simulink model "simulator"  (Simulink 7.3)
settings: Solver=ode1  SolverMode=SingleTasking  StartTime=0.0  StopTime=4  FixedStep=0.001  RelTol=1e-3
values from neighbouring files (symbols this model uses):
  Beq = 0.0015*6    (= 0.009)    [Sve ikad.m]    (also in matlab.mat = 0.0075)
  Eff_G = 0.9    [Sve ikad.m]    (also in matlab.mat)
  Eff_M = 0.69    [Sve ikad.m]    (also in matlab.mat)
  Jeq = 2e-3    (= 0.002)    [Sve ikad.m]    (also in matlab.mat)
  Ke = 0.0076776    [Sve ikad.m]    (also in matlab.mat)
  Kg = 70    [Sve ikad.m]    (also in matlab.mat)
  Km = 0.007683    [Sve ikad.m]    (also in matlab.mat)
  Ra = 2.6    [Sve ikad.m]    (also in matlab.mat)
settings Model: Creator=Labos  LastModifiedBy=Mehatronicki Sustavi

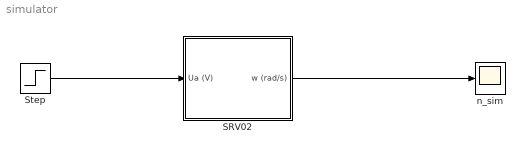
== system simulator ==
  "SRV02 " : Subsystem
  Step : Step
  n_sim : Scope
      settings: TimeRange=5  YMin=0  YMax=30  SaveName=n_sim  DataFormat=Array  SampleInput=on
  wires:
  Step/1 -> "SRV02 "/1(Ua (V))
  "SRV02 "/1(w (rad/s)) -> n_sim/1

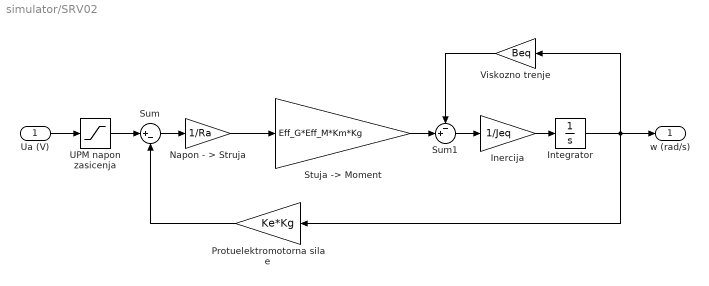
== system simulator/SRV02  ==
  Ua (V) : Inport
  Inercija : Gain  Gain=1/Jeq
  Integrator : Integrator
  Napon - > Struja : Gain  Gain=1/Ra
  Protuelektromotorna sila e : Gain  Gain=Ke*Kg
  "Stuja -> Moment" : Gain  Gain=Eff_G*Eff_M*Km*Kg
  Sum : Sum  Inputs=|+-
  Sum1 : Sum  Inputs=-+|
  UPM napon zasicenja : Saturate  UpperLimit=6  LowerLimit=-6
  Viskozno trenje : Gain  Gain=Beq
  w (rad/s) : Outport
  wires:
  Sum1/1 -> Inercija/1
  "Stuja -> Moment"/1 -> Sum1/2
  Inercija/1 -> Integrator/1
  UPM napon zasicenja/1 -> Sum/1
  Napon - > Struja/1 -> "Stuja -> Moment"/1
  Ua (V)/1 -> UPM napon zasicenja/1
  Sum/1 -> Napon - > Struja/1
  Viskozno trenje/1 -> Sum1/1
  Protuelektromotorna sila e/1 -> Sum/2
  Integrator/1 -> w (rad/s)/1, Protuelektromotorna sila e/1, Viskozno trenje/1
